simulink model "TH3_7m"  (R2018b)
settings: Solver=VariableStepAuto  StartTime=0.0  StopTime=100  RelTol=1e-3
values from neighbouring files (symbols this model uses):
  k = place(A, B, poles)    [PCA_6.m]    (also in TH3_7.m; TH3_8.m)
settings Model: Creator=ohara  LastModifiedBy=ohara

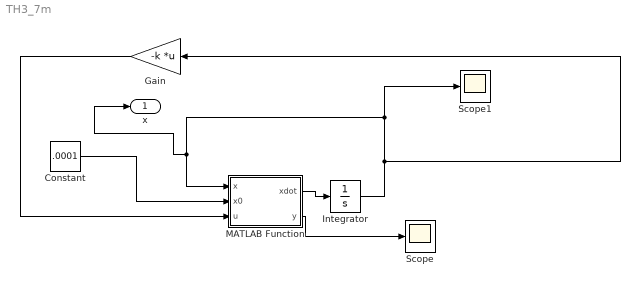
== system TH3_7m ==
  Constant : Constant  Value=.0001
  Gain : Gain  Gain=-k  Multiplication=Matrix(K*u)
  Integrator : Integrator  InitialCondition=[3,3,0]
  MATLAB Function : MATLAB Function  TreatAsAtomicUnit=on
  Scope : Scope
  Scope1 : Scope
  x : Outport
  wires:
  Integrator/1 -> Scope1/1, x/1, MATLAB Function/1(x), Gain/1
  MATLAB Function/1(xdot) -> Integrator/1
  MATLAB Function/2(y) -> Scope/1
  Constant/1 -> MATLAB Function/2(x0)
  Gain/1 -> MATLAB Function/3(u)

== matlab function TH3_7m/MATLAB Function ==
  data: x input; x0 input; xdot output; u input; y output
function [xdot, y] = TH3(x, x0, u)
xdot1 = -3*x(1) +   x(2) + u;
xdot2 =    x(1) - 2*x(2) - x(3);
xdot3 =    x(2) - 3*x(3) + x0;
xdot  =   [xdot1 ; xdot2 ; xdot3];
y     =    x(3);
